simulink model "untitled"  (R2020a)
settings: Solver=VariableStepAuto  StartTime=0.0  StopTime=10.0  RelTol=1e-3
undefined symbols (not defined in the file or in its folder): sigbuilder_block
settings Model: Creator=Jason  LastModifiedBy=Jason

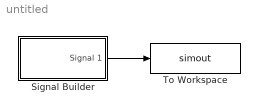
== system untitled ==
  Signal Builder : Subsystem  Tag=STV Subsys  LoadFcn=sigbuilder_block('load',[0 22.5 1440 729.75 ]);  StartFcn=sigbuilder_block('start');  StopFcn=sigbuilder_block('stop');  ClipboardFcn=sigbuilder_block('clipboard');  mask(Sigbuilder block){tuvar=[0:10]}
      mask help: Simulink:masks:SigbuilderBlock_MD
      mask init:
      | if ~strcmp(get_param(bdroot(gcbh),'SimulationStatus'),'stopped') tuvar = sigbuilder_block('maskInit'); end
      settings: CopyFcn=sigbuilder_block('copy');  DeleteFcn=sigbuilder_block('delete');  ModelCloseFcn=sigbuilder_block('modelClose');  PreSaveFcn=sigbuilder_block('preSave');  PauseFcn=sigbuilder_block('pause');  ContinueFcn=sigbuilder_block('continue');  NameChangeFcn=sigbuilder_block('namechange');  OpenFcn=sigbuilder_block('open',[437.6 199.2 550.4 400 ]);  CloseFcn=sigbuilder_block('close');
      mask Display: plot(0, 0, 100, 100,[2, 2, 32, 32, 2], [68, 8, 8, 68, 68],[32, 2], [38, 38], [32, 19, 2],[53, 60, 44], [32, 17, 17, 2],[16, 16, 31, 31]);txt = getActiveGroup(gcbh);text(2, 100, txt,'verticalAlignment', 'top');
  To Workspace : ToWorkspace  VariableName=simout  SaveFormat=Timeseries  SampleTime=-1
  wires:
  Signal Builder/1(Signal 1) -> To Workspace/1

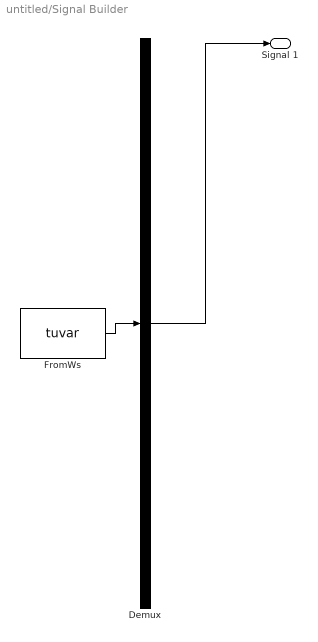
== system untitled/Signal Builder ==
  Demux : Demux  Tag=STV Demux  Outputs=1
      settings: DisplayOption=none
  FromWs : FromWorkspace  Tag=STV FromWs  VariableName=tuvar
      SigBuilderData=|
      | common.afterFinalStr = 'Extrapolate'
      | common.sampleTime = 0
      | dataSet.timeRange = [0 10]
      | dataSet.name = 'Group 1'
      | sbobj.Groups.Name = 'Group 1'
      | sbobj.Groups.Signals.Name = 'Signal 1'
      | sbobj.Groups.Signals.XData = [0 0.1 0.2 0.32 0.44 0.56 0.68 0.96 1.1 1.24 1.36 1.5 1.62 1.72 1.86 1.98 2.1 2.22 2.34 2.48 2.6 2.72 2.84 2.98 3.12 3.24 3.38 3.5 3.64 3.74 3.84 3.98 4.08 4.22 4.32 4.48 4.6 4.74 4.88 4.98 5.12 5.26 5.36 5.5 5.62 5.74 5.84 5.98 6.1 6.22 6.32 6.48 6.58 6.74 6.86 6.98 7.12 7.24 7.34 7.46 7.6 7.72 7.85 7.98 8.08 8.18 8.31 8.44 8.55 8.7 8.82 8.98 9.08 9.2 9.31 9.46 9.58 9.72 9.87 10]
      | sbobj.Groups.Signals.YData = [-0.04 -0.232 -0.444 -0.676 -0.89 -0.914 -0.942 -1 -0.996 -0.996 -0.994 -0.992 -0.958 -0.928 -0.89 -0.856 -0.78 -0.688 -0.608 -0.5 -0.458 -0.416 -0.376 -0.33 -0.296 -0.262 -0.23 -0.198 -0.184 -0.17 -0.16 -0.144 -0.136 -0.124 -0.116 -0.104 -0.1 -0.094 -0.092 -0.088 -0.084 -0.078 -0.076 -0.072 -0.068 -0.062 -0.06 -0.054 -0.05 -0.046 -0.044 -0.038 -0.036 -0.032 -0.03 -0.026 -0.024 -0.02 -0.018 -0.014 -0.0129230769231 -0.012 -0.011 -0.01 -0.009 -0.008 -0.008 -0.008 -0.00715384615385 -0.006 -0.006 -0.006 -0.00509090909091 -0.004 -0.00315384615385 -0.002 -0.00107692307692 0 0 0]
      | sbobj.Groups.TimeRange = [0 1000]
  Signal 1 : Outport  Tag=STV Outport
  wires:
  Demux/1 -> Signal 1/1
  FromWs/1 -> Demux/1
